simulink library "explorerHatPro"  (R2021b)
settings: Solver=VariableStepAuto  StartTime=0.0  StopTime=10.0  RelTol=1e-3
libraries: raspberrypiBasiclib x12, simulink x8, raspberrypiCommlib x3
settings Model: Creator=ebene  LastModifiedBy=ebene

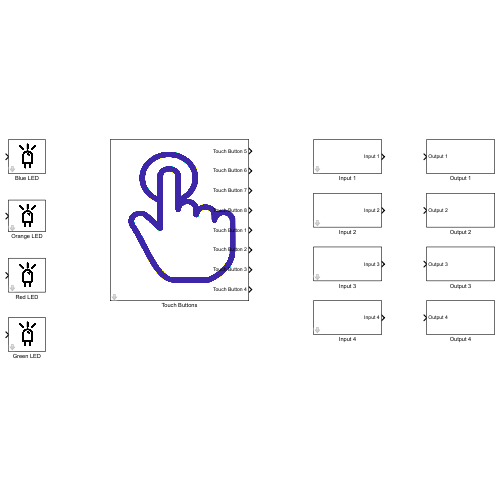
[thumbnail: Simulink's stored preview of the top-level diagram]
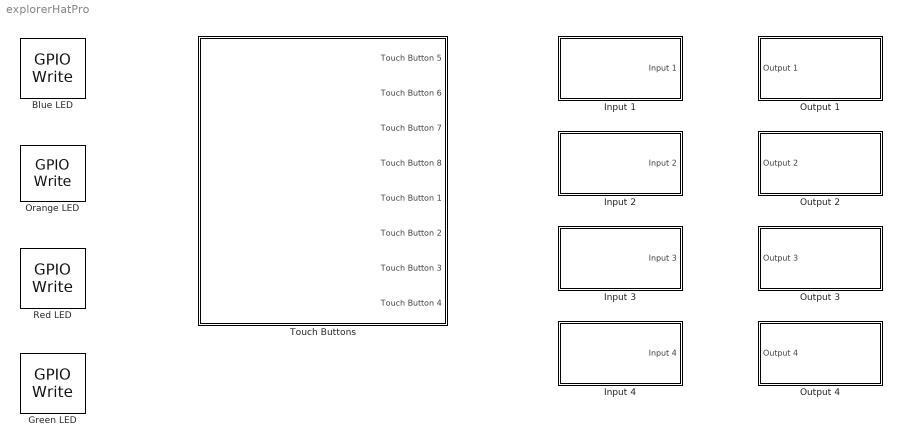
== system explorerHatPro ==
  Blue LED : raspberrypiBasiclib/GPIO Write  board=Pi 4 Model B  gpio=4  direction=Output  blockPlatform=Raspberry Pi  mask(GPIO Write){}
      settings: SourceProductBaseCode=RASPPI
      mask Display:
      | % This is a new mask on top of the base mask.
      | % Use "View base mask" link below to see the base mask.
      | image(imread('./src/ExplorerHat/icons/LED.png'))
  Green LED : raspberrypiBasiclib/GPIO Write  board=Pi 4 Model B  gpio=5  direction=Output  blockPlatform=Raspberry Pi  mask(GPIO Write){}
      settings: SourceProductBaseCode=RASPPI
      mask Display:
      | % This is a new mask on top of the base mask.
      | % Use "View base mask" link below to see the base mask.
      | image(imread('./src/ExplorerHat/icons/LED.png'))
  Input 1 : Subsystem  mask{SampleTime=0.01}
      mask prompts: SampleTime "Sample Time"
  Input 2 : Subsystem  mask{SampleTime=0.01}
      mask prompts: SampleTime "Sample Time"
  Input 3 : Subsystem  mask{SampleTime=0}
      mask prompts: SampleTime "Sample Time"
  Input 4 : Subsystem  mask{SampleTime=0.01}
      mask prompts: SampleTime "Sample Time"
  Orange LED : raspberrypiBasiclib/GPIO Write  board=Pi 4 Model B  gpio=17  direction=Output  blockPlatform=Raspberry Pi  mask(GPIO Write){}
      settings: SourceProductBaseCode=RASPPI
      mask Display:
      | % This is a new mask on top of the base mask.
      | % Use "View base mask" link below to see the base mask.
      | image(imread('./src/ExplorerHat/icons/LED.png'))
  Output 1 : Subsystem
  Output 2 : Subsystem
  Output 3 : Subsystem
  Output 4 : Subsystem
  Red LED : raspberrypiBasiclib/GPIO Write  board=Pi 4 Model B  gpio=27  direction=Output  blockPlatform=Raspberry Pi  mask(GPIO Write){}
      settings: SourceProductBaseCode=RASPPI
      mask Display:
      | % This is a new mask on top of the base mask.
      | % Use "View base mask" link below to see the base mask.
      | image(imread('./src/ExplorerHat/icons/LED.png'))
  Touch Buttons : Subsystem  mask{SampleTime=0.01}
      mask prompts: SampleTime "Sample Time"
      mask Display: image(imread('./src/ExplorerHat/icons/touchButton.png'));

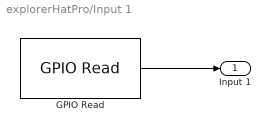
== system explorerHatPro/Input 1 ==
  GPIO Read : raspberrypiBasiclib/GPIO Read  board=Pi 4 Model B  gpio=23  internalResistor=Off  sampleTime=SampleTime  direction=Input  blockPlatform=Raspberry Pi
      settings: SourceProductBaseCode=RASPPI
  Input 1 : Outport
  wires:
  GPIO Read/1 -> Input 1/1

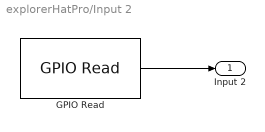
== system explorerHatPro/Input 2 ==
  GPIO Read : raspberrypiBasiclib/GPIO Read  board=Pi 4 Model B  gpio=22  internalResistor=Off  sampleTime=SampleTime  direction=Input  blockPlatform=Raspberry Pi
      settings: SourceProductBaseCode=RASPPI
  Input 2 : Outport
  wires:
  GPIO Read/1 -> Input 2/1

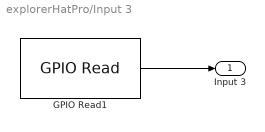
== system explorerHatPro/Input 3 ==
  GPIO Read1 : raspberrypiBasiclib/GPIO Read  board=Pi 4 Model B  gpio=24  internalResistor=Off  sampleTime=SampleTime  direction=Input  blockPlatform=Raspberry Pi
      settings: SourceProductBaseCode=RASPPI
  Input 3 : Outport
  wires:
  GPIO Read1/1 -> Input 3/1

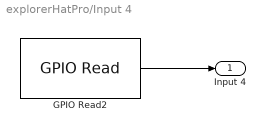
== system explorerHatPro/Input 4 ==
  GPIO Read2 : raspberrypiBasiclib/GPIO Read  board=Pi 4 Model B  gpio=25  internalResistor=Off  sampleTime=SampleTime  direction=Input  blockPlatform=Raspberry Pi
      settings: SourceProductBaseCode=RASPPI
  Input 4 : Outport
  wires:
  GPIO Read2/1 -> Input 4/1

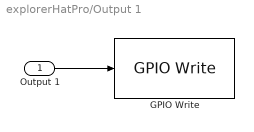
== system explorerHatPro/Output 1 ==
  Output 1 : Inport
  GPIO Write : raspberrypiBasiclib/GPIO Write  board=Pi 4 Model B  gpio=6  direction=Output  blockPlatform=Raspberry Pi
      settings: SourceProductBaseCode=RASPPI
  wires:
  Output 1/1 -> GPIO Write/1

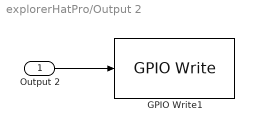
== system explorerHatPro/Output 2 ==
  Output 2 : Inport
  GPIO Write1 : raspberrypiBasiclib/GPIO Write  board=Pi 4 Model B  gpio=12  direction=Output  blockPlatform=Raspberry Pi
      settings: SourceProductBaseCode=RASPPI
  wires:
  Output 2/1 -> GPIO Write1/1

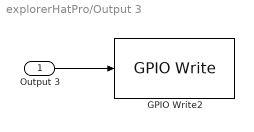
== system explorerHatPro/Output 3 ==
  Output 3 : Inport
  GPIO Write2 : raspberrypiBasiclib/GPIO Write  board=Pi 4 Model B  gpio=13  direction=Output  blockPlatform=Raspberry Pi
      settings: SourceProductBaseCode=RASPPI
  wires:
  Output 3/1 -> GPIO Write2/1

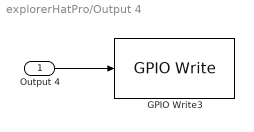
== system explorerHatPro/Output 4 ==
  Output 4 : Inport
  GPIO Write3 : raspberrypiBasiclib/GPIO Write  board=Pi 4 Model B  gpio=16  direction=Output  blockPlatform=Raspberry Pi
      settings: SourceProductBaseCode=RASPPI
  wires:
  Output 4/1 -> GPIO Write3/1

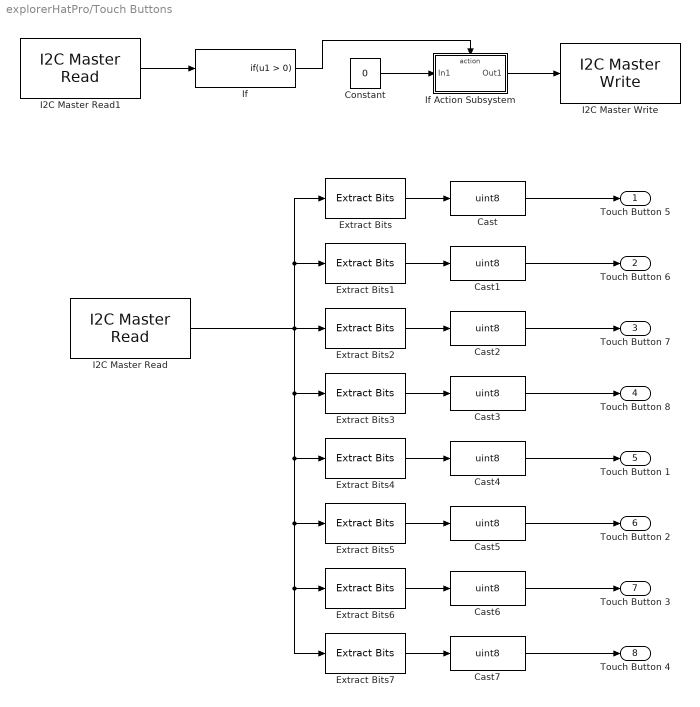
== system explorerHatPro/Touch Buttons ==
  Cast{,1..7} (8 alike) : DataTypeConversion  OutMin=[0]  OutMax=[128]  OutDataTypeStr=uint8
  Constant : Constant  Value=0  OutDataTypeStr=uint8
  Extract Bits : simulink/Logic and Bit Operations/Extract Bits  bitsToExtract=Range of bits  numBits=8  bitIdxRange=[0]  outScalingMode=Preserve fixed-point scaling
  Extract Bits1 : simulink/Logic and Bit Operations/Extract Bits  bitsToExtract=Range of bits  numBits=8  bitIdxRange=[1]  outScalingMode=Preserve fixed-point scaling
  Extract Bits2 : simulink/Logic and Bit Operations/Extract Bits  bitsToExtract=Range of bits  numBits=8  bitIdxRange=[2]  outScalingMode=Preserve fixed-point scaling
  Extract Bits3 : simulink/Logic and Bit Operations/Extract Bits  bitsToExtract=Range of bits  numBits=8  bitIdxRange=[3]  outScalingMode=Preserve fixed-point scaling
  Extract Bits4 : simulink/Logic and Bit Operations/Extract Bits  bitsToExtract=Range of bits  numBits=8  bitIdxRange=[4]  outScalingMode=Preserve fixed-point scaling
  Extract Bits5 : simulink/Logic and Bit Operations/Extract Bits  bitsToExtract=Range of bits  numBits=8  bitIdxRange=[5]  outScalingMode=Preserve fixed-point scaling
  Extract Bits6 : simulink/Logic and Bit Operations/Extract Bits  bitsToExtract=Range of bits  numBits=8  bitIdxRange=[6]  outScalingMode=Preserve fixed-point scaling
  Extract Bits7 : simulink/Logic and Bit Operations/Extract Bits  bitsToExtract=Range of bits  numBits=8  bitIdxRange=[7]  outScalingMode=Preserve fixed-point scaling
  I2C Master Read : raspberrypiCommlib/I2C Master Read  BoardProperty=Pi 4 Model B  Mode=Master  SlaveAddress=hex2dec('28')  SlaveByteOrder=BigEndian  Direction=Receiver  RegisterAddressMode=on  RegisterAddress=3  SlaveDataType=uint8  DataLength=1  NoAck=off  RepeatedStart=off  OutputStatus=off  SampleTime=SampleTime
      settings: SourceProductBaseCode=RASPPI
  I2C Master Read1 : raspberrypiCommlib/I2C Master Read  BoardProperty=Pi 4 Model B  Mode=Master  SlaveAddress=hex2dec('28')  SlaveByteOrder=BigEndian  Direction=Receiver  RegisterAddressMode=on  RegisterAddress=0  SlaveDataType=uint8  DataLength=1  NoAck=off  RepeatedStart=off  OutputStatus=off  SampleTime=SampleTime
      settings: SourceProductBaseCode=RASPPI
  I2C Master Write : raspberrypiCommlib/I2C Master Write  BoardProperty=Pi 4 Model B  Mode=Master  SlaveAddress=hex2dec('28')  SlaveByteOrder=BigEndian  Direction=Transmitter  RegisterAddressMode=on  RegisterAddress=0  SlaveDataType=uint8  DataLength=1  NoAck=off  RepeatedStart=off  OutputStatus=off
      settings: SourceProductBaseCode=RASPPI
  If : If  ShowElse=off
  If Action Subsystem : Subsystem  TreatAsAtomicUnit=on
  Touch Button 5 : Outport
  Touch Button 6 : Outport  Port=2
  Touch Button 7 : Outport  Port=3
  Touch Button 8 : Outport  Port=4
  Touch Button 1 : Outport  Port=5
  Touch Button 2 : Outport  Port=6
  Touch Button 3 : Outport  Port=7
  Touch Button 4 : Outport  Port=8
  wires:
  I2C Master Read/1 -> Extract Bits4/1, Extract Bits5/1, Extract Bits6/1, Extract Bits7/1, Extract Bits3/1, Extract Bits/1, Extract Bits1/1, Extract Bits2/1
  Extract Bits/1 -> Cast/1
  Extract Bits3/1 -> Cast3/1
  Extract Bits6/1 -> Cast6/1
  Extract Bits7/1 -> Cast7/1
  Extract Bits1/1 -> Cast1/1
  If Action Subsystem/1(Out1) -> I2C Master Write/1
  Extract Bits2/1 -> Cast2/1
  Extract Bits5/1 -> Cast5/1
  If/1 -> If Action Subsystem/Action
  I2C Master Read1/1 -> If/1
  Constant/1 -> If Action Subsystem/1(In1)
  Cast3/1 -> Touch Button 8/1
  Cast5/1 -> Touch Button 2/1
  Extract Bits4/1 -> Cast4/1
  Cast2/1 -> Touch Button 7/1
  Cast4/1 -> Touch Button 1/1
  Cast1/1 -> Touch Button 6/1
  Cast7/1 -> Touch Button 4/1
  Cast6/1 -> Touch Button 3/1
  Cast/1 -> Touch Button 5/1

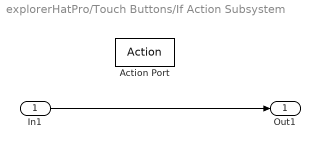
== system explorerHatPro/Touch Buttons/If Action Subsystem ==
  In1 : Inport
  Action Port : ActionPort  ActionPortLabel=if(u1 > 0)
  Out1 : Outport
  wires:
  In1/1 -> Out1/1
